simulink model "sim_ekf_est_all_para_v2"  (R2020b)
settings: Solver=ode1  StartTime=0.0  StopTime=20  FixedStep=0.01  RelTol=1e-3
settings Model: Creator=Admin  LastModifiedBy=ONLY-GOD

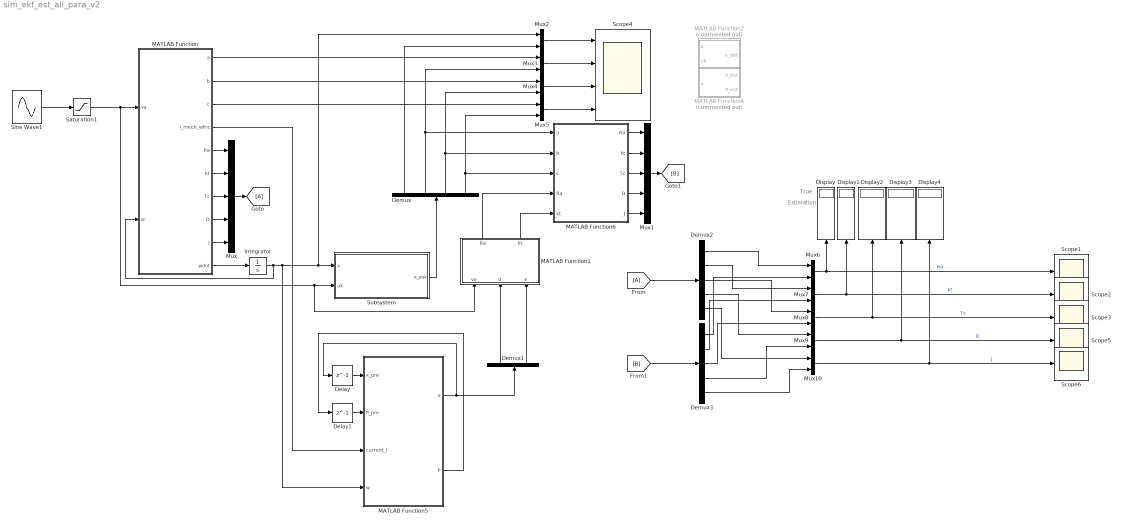
== system sim_ekf_est_all_para_v2 ==
  note: Estimation
  note: True
  Delay : Delay  DelayLength=1  InitialCondition=[0.01,0.01]
  Delay1 : Delay  DelayLength=1  InitialCondition=1e-5*eye(2)
  Demux : Demux
  Demux1 : Demux  Outputs=2
  Demux2 : Demux  Outputs=5
  Demux3 : Demux  Outputs=5
  Display{,1..4} (5 alike) : Display
  Integrator : Integrator
  MATLAB Function : MATLAB Function  TreatAsAtomicUnit=on
  MATLAB Function1 : MATLAB Function  TreatAsAtomicUnit=on
  MATLAB Function2 : MATLAB Function  Commented=on  TreatAsAtomicUnit=on
  MATLAB Function4 : MATLAB Function  Commented=on  TreatAsAtomicUnit=on
  MATLAB Function5 : MATLAB Function  TreatAsAtomicUnit=on
  MATLAB Function6 : MATLAB Function  TreatAsAtomicUnit=on
  Mux : Mux  Inputs=5
  Mux1 : Mux  Inputs=5
  Mux{2..10} (9 alike) : Mux  Inputs=2
  Saturation1 : Saturate  UpperLimit=24  LowerLimit=-24
  Scope{1..3,5..6} (5 alike) : Scope
  Scope4 : Scope  NumInputPorts=4
  Sine Wave1 : Sin  Amplitude=6  Frequency=2*pi*1  SampleTime=0
  Subsystem : Subsystem
  wires:
  MATLAB Function/2(b) -> Mux4/1
  MATLAB Function/4(i_mech_wfric) -> MATLAB Function5/3(current_i)
  Sine Wave1/1 -> Saturation1/1
  Saturation1/1 -> MATLAB Function1/1(va), Subsystem/2(uk), MATLAB Function/1(va)
  MATLAB Function/3(c) -> Mux5/1
  MATLAB Function/10(wdot) -> Integrator/1
  MATLAB Function/1(a) -> Mux3/1
  Integrator/1 -> Mux2/1, Subsystem/1(x), MATLAB Function5/4(w), MATLAB Function/2(w)
  Mux2/1 -> Scope4/1
  Mux3/1 -> Scope4/2
  Mux4/1 -> Scope4/3
  Mux5/1 -> Scope4/4
  Demux/1 -> Mux2/2
  Demux/2 -> Mux3/2, MATLAB Function6/1(a)
  Demux/3 -> Mux4/2, MATLAB Function6/2(b)
  Demux/4 -> Mux5/2, MATLAB Function6/3(c)
  Delay/1 -> MATLAB Function5/1(x_pre)
  Delay1/1 -> MATLAB Function5/2(P_pre)
  MATLAB Function5/1(x) -> Delay/1, Demux1/1
  MATLAB Function5/2(P) -> Delay1/1
  Subsystem/1(x_est) -> Demux/1
  MATLAB Function/5(Ra) -> Mux/1
  MATLAB Function/6(kt) -> Mux/2
  MATLAB Function/7(Tc) -> Mux/3
  MATLAB Function/8(D) -> Mux/4
  MATLAB Function/9(J) -> Mux/5
  MATLAB Function6/1(Ra) -> Mux1/1
  MATLAB Function6/2(kt) -> Mux1/2
  MATLAB Function6/3(Tc) -> Mux1/3
  MATLAB Function6/4(D) -> Mux1/4
  MATLAB Function6/5(J) -> Mux1/5
  Mux/1 -> [A]
  Mux1/1 -> [B]
  Mux6/1 -> Display/1, Scope1/1  "Ra"
  Mux7/1 -> Display1/1, Scope2/1  "kt"
  Mux8/1 -> Scope3/1, Display2/1  "Tc"
  Mux9/1 -> Display3/1, Scope5/1  "D"
  Mux10/1 -> Display4/1, Scope6/1  "J"
  [A] -> Demux2/1
  [B] -> Demux3/1
  Demux2/1 -> Mux6/1
  Demux2/2 -> Mux7/1
  Demux2/3 -> Mux8/1
  Demux2/4 -> Mux9/1
  Demux2/5 -> Mux10/1
  Demux3/1 -> Mux6/2
  Demux3/2 -> Mux7/2
  Demux3/3 -> Mux8/2
  Demux3/4 -> Mux9/2
  Demux3/5 -> Mux10/2
  MATLAB Function1/1(Ra) -> MATLAB Function6/4("Ra ")
  MATLAB Function1/2(kt) -> MATLAB Function6/5("kt ")
  Demux1/1 -> MATLAB Function1/2(d)
  Demux1/2 -> MATLAB Function1/3(e)

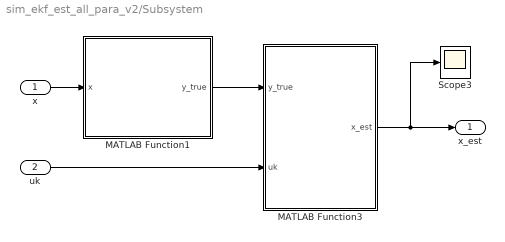
== system sim_ekf_est_all_para_v2/Subsystem ==
  x : Inport
  uk : Inport  Port=2
  MATLAB Function1 : MATLAB Function  TreatAsAtomicUnit=on
  MATLAB Function3 : MATLAB Function  TreatAsAtomicUnit=on
  Scope3 : Scope
  x_est : Outport
  wires:
  MATLAB Function1/1(y_true) -> MATLAB Function3/1(y_true)
  MATLAB Function3/1(x_est) -> Scope3/1, x_est/1
  uk/1 -> MATLAB Function3/2(uk)
  x/1 -> MATLAB Function1/1(x)

== matlab function sim_ekf_est_all_para_v2/Subsystem/MATLAB Function1 ==
  settings: updateMethod=DISCRETE
  data: x input; y_true output
function y_true = output_eq(x)
x = [x;0;0;0];
C = [1 0 0 0];
y_true = C*x;

== matlab function sim_ekf_est_all_para_v2/MATLAB Function ==
  settings: updateMethod=DISCRETE
  data: a output; b output; c output; i_mech_wfric output; Ra output; kt output; Tc output; D output; J output; va input; wdot output; w input
function [a,b,c,i_mech_wfric,Ra,kt,Tc,D,J,wdot] = fcn(va,w)
%parameters from datasheet
Ra = 14.3;
kt = 0.05; %kb = 0.063;
kb = kt;
Tc = 0.053*kt;
D  = 9.4e-5*kt;
J = 1.94e-4*kt;

% lumped parameters
a = ((kb*kt+D*Ra)/(Ra*J));
b = (kt/(Ra*J));
c = (Tc/J);

% model
wdot = -a*w + b*va - c*sign(w);

% i_elec = (va - kb*w)/Ra;
% i_mech_nfric = (D*w + J*wdot)/kt;
i_mech_wfric = (Tc*sign(w)+0.001*randn+D*w + J*wdot)/kt;

== matlab function sim_ekf_est_all_para_v2/MATLAB Function2 ==
  data: x input; x_dot output; uk input
function x_dot = state_eq(x,uk)
x_dot = [0;0;0;0];
x_dot(1) = -x(1)*x(2)+x(3)*uk+sqrt(0.02)-x(4)*sign(x(1))*sqrt(0.01)*randn;
x_dot(2) = 0;
x_dot(3) = 0;
x_dot(4) = 0;

== matlab function sim_ekf_est_all_para_v2/MATLAB Function4 ==
  data: u input; x_est output; P_est output
function [x_est,P_est] = fcn(u)
Ts = 0.01;
persistent x_est_p P_est_p Qd_est R_est Qc_est;
if isempty(x_est_p)
    x_est_p = [0;0];
    P_est_p = 1e0*diag([10,1]);
    Qc_est  = 1e-4*diag([1,10]);
    Qd_est  = Ts*Qc_est;
    R_est   = 0.001;
end
A = [1 0;0 1];
B = [0 ; 0];
C = [i -w];
D = 0;

% Time Update
x_est = x_est_p;
P_est = A*P_est_p*A' + Qd_est;

% Measurement Update
va_est = C*x_est;
Pxy = P_est*C';
Pyy = C*P_est*C' + R_est;
W = Pxy*Pyy';
x_est = x_est + W*(va_input - va_est);
P_est = P_est - W*Pyy*W';

== matlab function sim_ekf_est_all_para_v2/Subsystem/MATLAB Function3 ==
  settings: updateMethod=DISCRETE
  data: y_true input; x_est output; uk input
function x_est = ekf(y_true, uk)
Ts = 0.01;
persistent x_est_p P Qd_est R_est Qc_est;
if isempty(x_est_p)
    x_est_p = [0;0;0;0];
    P       = 1e0*diag([10,1,30,10]);
    Qc_est  = 1e-4*diag([1,10,100,10]);
    Qd_est  = Ts*Qc_est;
    R_est   = 0.001;
end
c  = [1 0 0 0];
D  = 0;
Ck = c;
Dk = D;

%Comput Kalman Gain and update predicted value
Wk    = P*Ck'/(Ck*P*Ck'+R_est);
y_est = Ck*x_est_p+Dk*uk;
x     = x_est_p+Wk.*(y_true-y_est);

%Compute prediction at next time step
x_est = x+Ts*[-x(2)*x(1)+uk*x(3)-x(4)*sign(x(1));
    0;
    0;
    0];

%Update error covariance matrices
P = P-Wk*Ck*P;

%Define Ak
Ak      = eye(4)+Ts*[-x(2) -x(1) uk -sign(x(1));
    0     0    0      0;
    0     0    0      0;
    0     0    0      0];
P       = Ak*P*Ak'+Qd_est;
x_est_p = x_est;

== matlab function sim_ekf_est_all_para_v2/MATLAB Function5 ==
  data: x_pre input; P_pre input; current_i input; x output; w input; P output
function [x,P] = kalman_omega(x_pre,P_pre,current_i,w)
% predefined
Ts = 0.01;
Q = 1e-1*diag([1 1]);
Qd = Q*Ts;
R = 1e-2;
% model prediction
A = [1 0;
     0 1];
B = [0;
     0];
C = [1 -w];

u = 0;

x = A*x_pre + B*u;
P = A*P_pre*A' + Qd;

%update
i_est = C*x;
er_i = current_i - i_est;
P_xy = P*C';
P_yy = C*P*C' + R;
x = x + (P_xy/P_yy)*er_i;
P = P - (P_xy/P_yy)*P_xy';

== matlab function sim_ekf_est_all_para_v2/MATLAB Function6 ==
  data: Ra output; kt output; Tc output; D output; a input; b input; c input; Ra input; J output; kt input
function [Ra,kt,Tc,D,J] = fcn(a,b,c,Ra,kt)
Ra = Ra;
kt = kt;

J = (kt/(Ra*b));
Tc = (c*J);
D = (a*Ra*J - kt^2)/Ra;

== matlab function sim_ekf_est_all_para_v2/MATLAB Function1 ==
  data: va input; d input; Ra output; e input; kt output
function [Ra,kt] = fcn(va,d,e)

Ra = va/d;
kt = e*Ra;
